simulink model "OMAP"  (R2018b)
settings: Solver=FixedStepDiscrete  StartTime=0.0  StopTime=10.0  FixedStep=0.01  RelTol=1e-3
values from neighbouring files (symbols this model uses):
  Clb_ICADirect_LaneDisp_StateFive = Simulink.Parameter    [omap_ver_442.m]
  Clb_ICADirect_LaneDisp_StateFour = Simulink.Parameter    [omap_ver_442.m]
  Clb_ICADirect_LaneDisp_StateOne = Simulink.Parameter    [omap_ver_442.m]
  Clb_ICADirect_LaneDisp_StateThree = Simulink.Parameter    [omap_ver_442.m]
  Clb_ICADirect_LaneDisp_StateTwo = Simulink.Parameter    [omap_ver_442.m]
  Clb_ICADirect_LaneDisp_StateZero = Simulink.Parameter    [omap_ver_442.m]
  Clb_ICADirect_LaneDispSW = Simulink.Parameter    [omap_ver_442.m]
  Clb_ICADirect_TrnLghtsCom_Switch = Simulink.Parameter    [omap_ver_442.m]
  Clb_ICADirect_TrnLghtsCom_Value = Simulink.Parameter    [omap_ver_442.m]
  Clb_ICADirect_TrnLghtsCrtl_Inhb = Simulink.Parameter    [omap_ver_442.m]
  OMAP_ACCAEB_EMSESC_Decel = Simulink.Parameter    [omap_ver_442.m]
  OMAP_ACCFCW_IC_Decel = Simulink.Parameter    [omap_ver_442.m]
  OMAP_clb_ACC_RVVReqType = Simulink.Parameter    [omap_ver_442.m]
  OMAP_clb_ACC_RVVReqType_Switch = Simulink.Parameter    [omap_ver_442.m]
  OMAP_clb_ACCHeadwayDisplay = Simulink.Parameter    [omap_ver_442.m]
  OMAP_clb_ACCHeadwayDisplay_Switch = Simulink.Parameter    [omap_ver_442.m]
  OMAP_clb_ACCHeadwayIcon = Simulink.Parameter    [omap_ver_442.m]
  OMAP_clb_ACCHeadwayIcon_Switch = Simulink.Parameter    [omap_ver_442.m]
  OMAP_clb_ACCMessagePrompt = Simulink.Parameter    [omap_ver_442.m]
  OMAP_clb_ACCMessagePrompt_Switch = Simulink.Parameter    [omap_ver_442.m]
  OMAP_clb_ACCRequestEPB = Simulink.Parameter    [omap_ver_442.m]
  OMAP_clb_ACCRequestEPB_Switch = Simulink.Parameter    [omap_ver_442.m]
  OMAP_clb_ACCSetSpeed = Simulink.Parameter    [omap_ver_442.m]
  OMAP_clb_ACCSetSpeed_Switch = Simulink.Parameter    [omap_ver_442.m]
  OMAP_clb_ACCSetSpeedDis = Simulink.Parameter    [omap_ver_442.m]
  OMAP_clb_ACCSetSpeedDis_Switch = Simulink.Parameter    [omap_ver_442.m]
  OMAP_clb_ACCState = Simulink.Parameter    [omap_ver_442.m]
  OMAP_clb_ACCState_Switch = Simulink.Parameter    [omap_ver_442.m]
  OMAP_clb_ACCStatusIconDis = Simulink.Parameter    [omap_ver_442.m]
  OMAP_clb_ACCStatusIconDis_Switch = Simulink.Parameter    [omap_ver_442.m]
  OMAP_clb_ACCTorqueReq = Simulink.Parameter    [omap_ver_442.m]
  OMAP_clb_ACCTorqueReq_Switch = Simulink.Parameter    [omap_ver_442.m]
  OMAP_clb_ADAS_State = Simulink.Parameter    [omap_ver_442.m]
  OMAP_clb_ADAS_State_Switch = Simulink.Parameter    [omap_ver_442.m]
  OMAP_clb_AEBAlertReq = Simulink.Parameter    [omap_ver_442.m]
  OMAP_clb_AEBAlertReq_Switch = Simulink.Parameter    [omap_ver_442.m]
  OMAP_clb_AEBBrakingProg = Simulink.Parameter    [omap_ver_442.m]
  OMAP_clb_AEBBrakingProg_Switch = Simulink.Parameter    [omap_ver_442.m]
  OMAP_clb_AEBFaultStatus = Simulink.Parameter    [omap_ver_442.m]
  OMAP_clb_AEBFaultStatus_Switch = Simulink.Parameter    [omap_ver_442.m]
  OMAP_clb_AEBMassageDisp = Simulink.Parameter    [omap_ver_442.m]
  OMAP_clb_AEBMassageDisp_Switch = Simulink.Parameter    [omap_ver_442.m]
  OMAP_clb_AEBState = Simulink.Parameter    [omap_ver_442.m]
  OMAP_clb_AEBState_Switch = Simulink.Parameter    [omap_ver_442.m]
  OMAP_clb_AEBSwitchStatus = Simulink.Parameter    [omap_ver_442.m]
  OMAP_clb_AEBSwitchStatus_Switch = Simulink.Parameter    [omap_ver_442.m]
  OMAP_clb_BrakeRequest = Simulink.Parameter    [omap_ver_442.m]
  OMAP_clb_BrakeRequest_Switch = Simulink.Parameter    [omap_ver_442.m]
  OMAP_clb_DecelerationSet = Simulink.Parameter    [omap_ver_442.m]
  OMAP_clb_DecelerationSet_Switch = Simulink.Parameter    [omap_ver_442.m]
  OMAP_clb_DecelerationType = Simulink.Parameter    [omap_ver_442.m]
  OMAP_clb_DecelerationType_Switch = Simulink.Parameter    [omap_ver_442.m]
  OMAP_clb_DeclControlReq = Simulink.Parameter    [omap_ver_442.m]
  OMAP_clb_DeclControlReq_Switch = Simulink.Parameter    [omap_ver_442.m]
  OMAP_clb_DownorUpGearMinTime = Simulink.Parameter    [omap_ver_442.m]
  OMAP_clb_DownorUpGearMinTime_Switch = Simulink.Parameter    [omap_ver_442.m]
  OMAP_clb_ELKPopupMessage = Simulink.Parameter    [omap_ver_442.m]
  OMAP_clb_ELKPopupMessage_Switch = Simulink.Parameter    [omap_ver_442.m]
  OMAP_clb_ELKSts = Simulink.Parameter    [omap_ver_442.m]
  OMAP_clb_ELKSts_Switch = Simulink.Parameter    [omap_ver_442.m]
  OMAP_clb_ESAFaultSt = Simulink.Parameter    [omap_ver_442.m]
  OMAP_clb_ESAFaultSt_Switch = Simulink.Parameter    [omap_ver_442.m]
  OMAP_clb_ESARequest = Simulink.Parameter    [omap_ver_442.m]
  OMAP_clb_ESARequest_Switch = Simulink.Parameter    [omap_ver_442.m]
  OMAP_clb_ESAState = Simulink.Parameter    [omap_ver_442.m]
  OMAP_clb_ESAState_Switch = Simulink.Parameter    [omap_ver_442.m]
  OMAP_clb_ESATorqueReq = Simulink.Parameter    [omap_ver_442.m]
  OMAP_clb_ESATorqueReq_Switch = Simulink.Parameter    [omap_ver_442.m]
  OMAP_clb_ESCDriveOff = Simulink.Parameter    [omap_ver_442.m]
  OMAP_clb_ESCDriveOff_Switch = Simulink.Parameter    [omap_ver_442.m]
  OMAP_clb_ESCHoldReq = Simulink.Parameter    [omap_ver_442.m]
  OMAP_clb_ESCHoldReq_Switch = Simulink.Parameter    [omap_ver_442.m]
  OMAP_clb_Handsoffwarning = Simulink.Parameter    [omap_ver_442.m]
  OMAP_clb_Handsoffwarning_Switch = Simulink.Parameter    [omap_ver_442.m]
  OMAP_clb_HapticAlarmReq = Simulink.Parameter    [omap_ver_442.m]
  OMAP_clb_HapticAlarmReq_Switch = Simulink.Parameter    [omap_ver_442.m]
  OMAP_clb_HMIPopupMassage = Simulink.Parameter    [omap_ver_442.m]
  OMAP_clb_HMIPopupMassage_Switch = Simulink.Parameter    [omap_ver_442.m]
  OMAP_clb_HWAActionSts = Simulink.Parameter    [omap_ver_442.m]
  OMAP_clb_HWAActionSts_Switch = Simulink.Parameter    [omap_ver_442.m]
  OMAP_clb_HWAMode = Simulink.Parameter    [omap_ver_442.m]
  OMAP_clb_HWAMode_Switch = Simulink.Parameter    [omap_ver_442.m]
  OMAP_clb_HWATurnOnIdctr = Simulink.Parameter    [omap_ver_442.m]
  OMAP_clb_HWATurnOnIdctr_Switch = Simulink.Parameter    [omap_ver_442.m]
  OMAP_clb_ICAMassageDisp = Simulink.Parameter    [omap_ver_442.m]
  OMAP_clb_ICAMassageDisp_Switch = Simulink.Parameter    [omap_ver_442.m]
  OMAP_clb_ICAStatusIcon = Simulink.Parameter    [omap_ver_442.m]
  OMAP_clb_ICAStatusIcon_Switch = Simulink.Parameter    [omap_ver_442.m]
  OMAP_clb_ISLCDriverRemind = Simulink.Parameter    [omap_ver_442.m]
  OMAP_clb_ISLCDriverRemind_Switch = Simulink.Parameter    [omap_ver_442.m]
  OMAP_clb_ISLCState = Simulink.Parameter    [omap_ver_442.m]
  OMAP_clb_ISLCState_Switch = Simulink.Parameter    [omap_ver_442.m]
  OMAP_clb_JAFaultSt = Simulink.Parameter    [omap_ver_442.m]
  OMAP_clb_JAFaultSt_Switch = Simulink.Parameter    [omap_ver_442.m]
  OMAP_clb_LCAPopupMessage = Simulink.Parameter    [omap_ver_442.m]
  OMAP_clb_LCAPopupMessage_Switch = Simulink.Parameter    [omap_ver_442.m]
  OMAP_clb_LCAStatusDisplay = Simulink.Parameter    [omap_ver_442.m]
  OMAP_clb_LCAStatusDisplay_Switch = Simulink.Parameter    [omap_ver_442.m]
  OMAP_clb_LDWStatusDisplay = Simulink.Parameter    [omap_ver_442.m]
  OMAP_clb_LDWStatusDisplay_Switch = Simulink.Parameter    [omap_ver_442.m]
  OMAP_clb_LDWWarningSt = Simulink.Parameter    [omap_ver_442.m]
  OMAP_clb_LDWWarningSt_Switch = Simulink.Parameter    [omap_ver_442.m]
  OMAP_clb_LightControlValid = Simulink.Parameter    [omap_ver_442.m]
  OMAP_clb_LightControlValid_Switch = Simulink.Parameter    [omap_ver_442.m]
  OMAP_clb_LKAActivation = Simulink.Parameter    [omap_ver_442.m]
  OMAP_clb_LKAActivation_Switch = Simulink.Parameter    [omap_ver_442.m]
  OMAP_clb_LKAAngleReq = Simulink.Parameter    [omap_ver_442.m]
  OMAP_clb_LKAAngleReq_Switch = Simulink.Parameter    [omap_ver_442.m]
  OMAP_clb_LKAMode = Simulink.Parameter    [omap_ver_442.m]
  OMAP_clb_LKAMode_Switch = Simulink.Parameter    [omap_ver_442.m]
  OMAP_clb_LKAorELK_CoolTime = Simulink.Parameter    [omap_ver_442.m]
  OMAP_clb_LKAState = Simulink.Parameter    [omap_ver_442.m]
  OMAP_clb_LKAState_Switch = Simulink.Parameter    [omap_ver_442.m]
  OMAP_clb_LKAStatusDisplay = Simulink.Parameter    [omap_ver_442.m]
  OMAP_clb_LKAStatusDisplay_Switch = Simulink.Parameter    [omap_ver_442.m]
  OMAP_clb_LKASwitchState = Simulink.Parameter    [omap_ver_442.m]
  OMAP_clb_LKASwitchState_Switch = Simulink.Parameter    [omap_ver_442.m]
  OMAP_clb_LKATorqFactReq = Simulink.Parameter    [omap_ver_442.m]
  OMAP_clb_LKATorqFactReq_Switch = Simulink.Parameter    [omap_ver_442.m]
  OMAP_clb_PrefillRequest = Simulink.Parameter    [omap_ver_442.m]
  ... (+36 more)
libraries: simulink x184, canmsglib x2
(part 12 of 14)

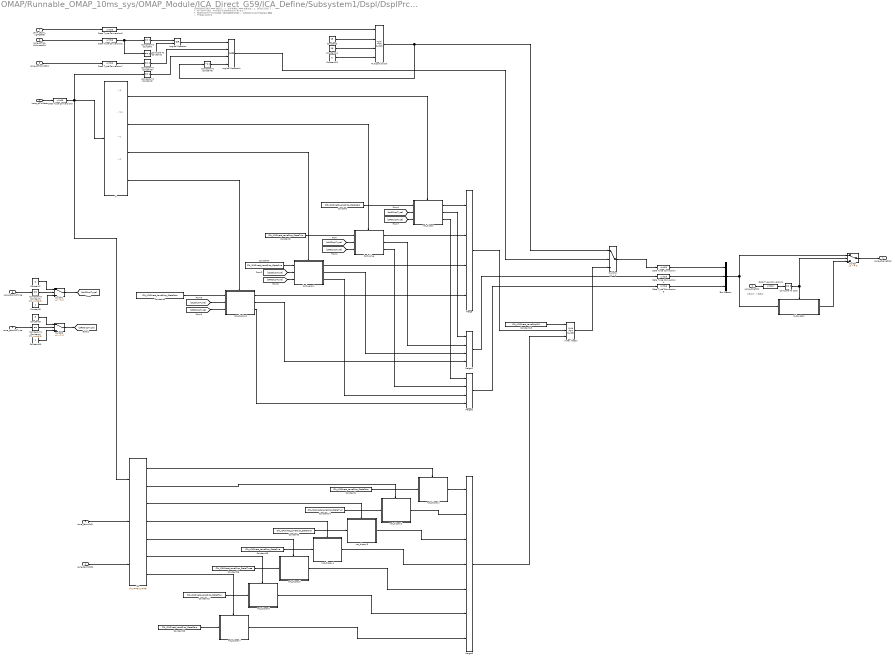
== system OMAP/Runnable_OMAP_10ms_sys/OMAP_Module/ICA_Direct_G59/ICA_Define/Subsystem1/Dspl/DsplPrcs/Lane ==
  note: 变道但条件不满足的车道线显示：
      | 1、多车道模式为TLC或者ALC；
      | 1、转向灯已经打了；
      | 2、由于条件不满足，THmode无法跳到状态4（=1或2）；
      | 3、驾驶员没有自己打方向变道（通过接管信号判断），此条其实可以由THState=3覆盖
      | 4、THState在状态3
  note: ->1
  note: ->14
  note: ->2
  note: ->0
  note: 0是运动，1是静止
  Lane_stTHState : Inport
  Lane_stVehSty : Inport  Port=2
  Lane_facmL0Ql : Inport  Port=3
  Lane_facmR0Ql : Inport  Port=4
  Lane_facmL0Type : Inport  Port=5
  Lane_facmR0Type : Inport  Port=6
  Lane_stturn_lightState : Inport  Port=7
  Lane_stTLC_ALCmodeSW : Inport  Port=8
  Lane_stTkOvStChk : Inport  Port=9
  Bus Creator : BusCreator  Inputs=3
  Compare To Constant : simulink/Logic and Bit Operations/Compare To Constant  relop===  const=2  OutDataTypeStr=boolean
  Compare To Constant1 : simulink/Logic and Bit Operations/Compare To Constant  relop===  const=3  OutDataTypeStr=boolean
  Compare To Constant2 : simulink/Logic and Bit Operations/Compare To Constant  relop===  const=3  OutDataTypeStr=boolean
  Compare To Constant3 : simulink/Logic and Bit Operations/Compare To Constant  relop===  const=uint16(3)  OutDataTypeStr=boolean
  Compare To Constant4 : simulink/Logic and Bit Operations/Compare To Constant  relop===  const=uint16(3)  OutDataTypeStr=boolean
  Compare To Constant5 : simulink/Logic and Bit Operations/Compare To Constant  relop===  const=0  OutDataTypeStr=boolean
  Compare To Constant6 : simulink/Logic and Bit Operations/Compare To Constant  relop=~=  const=0  OutDataTypeStr=boolean
  Compare To Zero : simulink/Logic and Bit Operations/Compare To Zero  relop===  OutDataTypeStr=boolean
  Constant{,1,5,13} (4 alike) : Constant  Value=Clb_ICADirect_LaneDisp_StateZero  OutDataTypeStr=uint16
  Constant10 : Constant  OutDataTypeStr=uint16
  Constant11 : Constant  Value=16  OutDataTypeStr=uint16
  Constant12 : Constant  Value=0  OutDataTypeStr=uint16
  Constant14 : Constant  Value=Clb_ICADirect_LaneDisp_StateTwo  OutDataTypeStr=uint16
  Constant15 : Constant  Value=Clb_ICADirect_LaneDisp_StateFive  OutDataTypeStr=uint16
  Constant16 : Constant  Value=Clb_ICADirect_LaneDisp_StateThree  OutDataTypeStr=uint16
  Constant17 : Constant  Value=Clb_ICADirect_LaneDisp_StateFour  OutDataTypeStr=uint16
  Constant18 : Constant  Value=Clb_ICADirect_LaneDispSW  OutDataTypeStr=boolean
  Constant2 : Constant  Value=Clb_ICADirect_LaneDisp_StateTwo  OutDataTypeStr=uint16
  Constant3 : Constant  Value=15  OutDataTypeStr=uint16
  Constant4 : Constant  Value=Clb_ICADirect_LaneDisp_StateOne  OutDataTypeStr=uint16
  Constant6 : Constant  Value=Clb_ICADirect_LaneDisp_StateOne  OutDataTypeStr=uint16
  Constant7 : Constant  Value=3  OutDataTypeStr=uint16
  Constant8 : Constant  OutDataTypeStr=uint16
  Constant9 : Constant  Value=3  OutDataTypeStr=uint16
  Data Type Conversion{,1..7} (8 alike) : DataTypeConversion  OutDataTypeStr=uint16
  If : If  IfExpression=u1==0|u1==5  ElseIfExpressions=u1==3,(u1==1|u1==2|u1==4|u1==6|u1==7|u1==8)
  If1 : If  NumInputs=3  IfExpression=u1==0|u1==5  ElseIfExpressions=u1==3,u1==1|u1==4|(u2<3&u3<3),u2==3&u3==3,u2==3&u3<3,u2<3&u3==3
  Index Vector : MultiPortSwitch  DataPortOrder=Zero-based contiguous  Inputs=2  zeroidx=on
  Logical Operator : Logic  Operator=OR  AllPortsSameDT=off  OutDataTypeStr=boolean
  Logical Operator1 : Logic  Inputs=4  AllPortsSameDT=off  OutDataTypeStr=boolean
  Merge : Merge  Inputs=4
  Merge1 : Merge  Inputs=4
  Merge2 : Merge  Inputs=4
  Merge3 : Merge  Inputs=7
  Multiport Switch : MultiPortSwitch  Inputs=2  DataPortIndices={1,2}  DataPortForDefault=Additional data port  DiagnosticForDefault=None
  Subsystem : Subsystem
  Switch : Switch  Criteria=u2 ~= 0
  Switch1 : Switch  Criteria=u2 ~= 0
  Switch2 : Switch  Criteria=u2 ~= 0
  Switch3 : Switch  Criteria=u2 > Threshold  OutDataTypeStr=uint16
  both_blue : Subsystem  TreatAsAtomicUnit=on
  both_gray1 : Subsystem  TreatAsAtomicUnit=on
  not_dispay : Subsystem  TreatAsAtomicUnit=on
  not_dispay1 : Subsystem  TreatAsAtomicUnit=on
  not_dispay2 : Subsystem  TreatAsAtomicUnit=on
  not_dispay3 : Subsystem  TreatAsAtomicUnit=on
  not_dispay4 : Subsystem  TreatAsAtomicUnit=on
  not_dispay5 : Subsystem  TreatAsAtomicUnit=on
  not_dispay6 : Subsystem  TreatAsAtomicUnit=on
  not_dispay7 : Subsystem  TreatAsAtomicUnit=on
  not_display2 : Subsystem  TreatAsAtomicUnit=on
  Lane_stLaneDspl : Outport
  wires:
  If/1 -> not_dispay/Action
  Lane_stVehSty/1 -> Data Type Conversion1/1
  both_gray1/1(Out1) -> Merge/3
  Lane_facmR0Type/1 -> Compare To Constant4/1
  Lane_facmR0Ql/1 -> If1/3
  Switch/1 -> Lane_stLaneDspl/1
  Compare To Zero/1 -> Switch/2, Subsystem/Enable
  Compare To Constant3/1 -> Switch1/2
  not_display2/1(Out1) -> Merge/4
  Lane_facmL0Type/1 -> Compare To Constant3/1
  Lane_facmL0Ql/1 -> If1/2
  Data Type Conversion5/1 -> Bus Creator/3  "stR0DispType"
  not_dispay/1(Out1) -> Merge/1
  [stL0DispType] -> both_blue/2(In2)
  Compare To Constant4/1 -> Switch2/2
  Constant2/1 -> both_blue/1(In1)
  both_blue/1(Out1) -> Merge/2
  Switch1/1 -> [stL0DispType]
  Subsystem/1(Out1) -> Switch/3
  [stR0DispType] -> both_blue/3(In3)
  Data Type Conversion4/1 -> Bus Creator/2  "stL0DispType"
  Constant8/1 -> Switch1/3
  Merge2/1 -> Data Type Conversion5/1
  Switch2/1 -> [stR0DispType]
  both_blue/3(Out3) -> Merge2/2
  Lane_stTHState/1 -> Data Type Conversion3/1
  Constant9/1 -> Switch2/1
  Merge1/1 -> Data Type Conversion4/1
  not_display2/3(Out3) -> Merge2/4
  Constant10/1 -> Switch2/3
  If/3 -> both_gray1/Action
  not_dispay/3(Out3) -> Merge2/1
  Constant7/1 -> Switch1/1
  If/2 -> both_blue/Action
  [stL0DispType] -> both_gray1/2(In2)
  If/4 -> not_display2/Action
  not_display2/2(Out2) -> Merge1/4
  Constant/1 -> not_dispay/1(In1)
  Bus Creator/1 -> Switch/1, Subsystem/1(In1)
  both_gray1/2(Out2) -> Merge1/3
  [stR0DispType] -> both_gray1/3(In3)
  Merge/1 -> Index Vector/2  "stLaneDspl"
  Data Type Conversion1/1 -> Compare To Zero/1
  [stR0DispType] -> not_dispay/3(In3)
  not_dispay/2(Out2) -> Merge1/1
  [stL0DispType] -> not_dispay/2(In2)
  [stL0DispType] -> not_display2/2(In2)
  Constant5/1 -> not_display2/1(In1)
  Constant4/1 -> both_gray1/1(In1)
  both_gray1/3(Out3) -> Merge2/3
  both_blue/2(Out2) -> Merge1/2
  [stR0DispType] -> not_display2/3(In3)
  Data Type Conversion/1 -> Bus Creator/1  "stLaneDspl"
  Switch3/1 -> Data Type Conversion/1
  Data Type Conversion2/1 -> Compare To Constant1/1, Compare To Constant/1
  Compare To Constant/1 -> Logical Operator/1
  Compare To Constant1/1 -> Logical Operator/2
  Lane_stTLC_ALCmodeSW/1 -> Data Type Conversion2/1
  Lane_stturn_lightState/1 -> Data Type Conversion6/1
  Lane_stTkOvStChk/1 -> Data Type Conversion7/1
  Data Type Conversion7/1 -> Compare To Constant5/1
  Constant3/1 -> Multiport Switch/2
  Constant11/1 -> Multiport Switch/3
  Constant12/1 -> Multiport Switch/4
  Data Type Conversion6/1 -> Multiport Switch/1
  Logical Operator/1 -> Logical Operator1/1
  Compare To Constant5/1 -> Logical Operator1/2
  Compare To Constant2/1 -> Logical Operator1/3
  Multiport Switch/1 -> Compare To Constant6/1, Switch3/1
  Compare To Constant6/1 -> Logical Operator1/4
  Logical Operator1/1 -> Switch3/2
  If1/1 -> not_dispay1/Action
  Constant1/1 -> not_dispay1/1(In1)
  Data Type Conversion3/1 -> If1/1, Compare To Constant2/1, If/1
  If1/2 -> not_dispay2/Action
  Constant14/1 -> not_dispay2/1(In1)
  If1/3 -> not_dispay3/Action
  Constant6/1 -> not_dispay3/1(In1)
  If1/4 -> not_dispay4/Action
  Constant15/1 -> not_dispay4/1(In1)
  If1/5 -> not_dispay5/Action
  Constant16/1 -> not_dispay5/1(In1)
  If1/6 -> not_dispay6/Action
  Constant17/1 -> not_dispay6/1(In1)
  If1/7 -> not_dispay7/Action
  Constant13/1 -> not_dispay7/1(In1)
  not_dispay1/1(Out1) -> Merge3/1
  not_dispay2/1(Out1) -> Merge3/2
  not_dispay3/1(Out1) -> Merge3/3
  not_dispay4/1(Out1) -> Merge3/4
  not_dispay5/1(Out1) -> Merge3/5
  not_dispay6/1(Out1) -> Merge3/6
  not_dispay7/1(Out1) -> Merge3/7
  Constant18/1 -> Index Vector/1
  Merge3/1 -> Index Vector/3  "stLaneDspl"
  Index Vector/1 -> Switch3/3

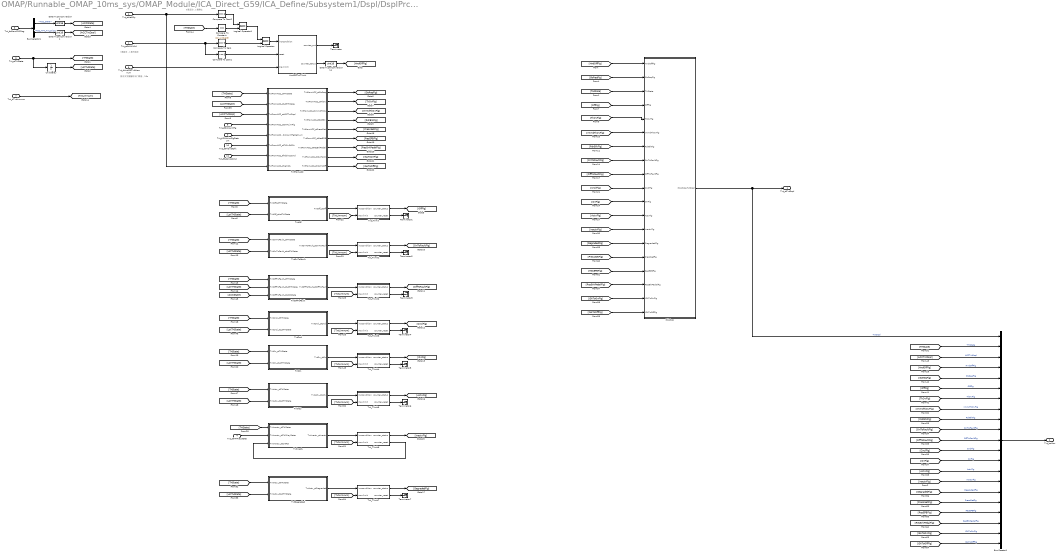
== system OMAP/Runnable_OMAP_10ms_sys/OMAP_Module/ICA_Direct_G59/ICA_Define/Subsystem1/Dspl/DsplPrcs/Txt ==
  note: 0是脱手，1是不脱手
  note: 脱手文字提醒时间门限值，15s
  note: 0是运动，1是静止
  Txt_stStWhlHld : Inport
  Txt_stVehSty : Inport  Port=2
  Txt_bsFromFMCMsg : Inport  Port=3
  Txt_stTHFKeyState : Inport  Port=4
  Txt_dHndOffTxtWarnnum : Inport  Port=5
  Txt_stTHState : Inport  Port=6
  Txt_dTxtLimnum : Inport  Port=7
  Txt_stSWALimFlg : Inport  Port=8
  Txt_tiSWALimFlgDetnum : Inport  Port=9
  Txt_stTkOvStChk : Inport  Port=10
  Txt_tfAddVocCmd : Inport  Port=11
  Bus Creator1 : BusCreator  Inputs=21
  Bus Selector1 : BusSelector  OutputSignals=ACC_State,ACC_HMI_Txt_Disp
  Compare To Constant : simulink/Logic and Bit Operations/Compare To Constant  relop===  const=uint16(3)  OutDataTypeStr=boolean
  Compare To Zero : simulink/Logic and Bit Operations/Compare To Zero  relop===  OutDataTypeStr=boolean
  Compare To Zero1 : simulink/Logic and Bit Operations/Compare To Zero  relop=~=  OutDataTypeStr=boolean
  Compare To Zero2 : simulink/Logic and Bit Operations/Compare To Zero  relop===  OutDataTypeStr=boolean
  Data Type Conversion1 : DataTypeConversion  OutDataTypeStr=uint16
  Data Type Conversion14 : DataTypeConversion  OutDataTypeStr=uint16
  Data Type Conversion2 : DataTypeConversion  OutDataTypeStr=uint16
  HndOffTxtTlimit : Subsystem
  Logical Operator : Logic  AllPortsSameDT=off  OutDataTypeStr=boolean
  Logical Operator1 : Logic  AllPortsSameDT=off  OutDataTypeStr=boolean
  PrioPrcs : MATLAB Function  TreatAsAtomicUnit=on
  Terminator{,1..7} (8 alike) : Terminator
  TxtActv : Subsystem
  TxtCncl : Subsystem
  TxtDegraded : Subsystem
  TxtFromACC : Subsystem
  TxtInactv : Subsystem
  TxtOff : Subsystem
  TxtOffToFault : Subsystem
  TxtOn : Subsystem
  TxtOnToFault : Subsystem
  Txt_Tlimit : Subsystem
  Txt_Tlimit1 : Subsystem
  Txt_Tlimit2 : Subsystem
  Txt_Tlimit3 : Subsystem
  Txt_Tlimit4 : Subsystem
  Txt_Tlimit5 : Subsystem
  Txt_Tlimit6 : Subsystem
  Txt_Tlimit7 : Subsystem
  Unit Delay : UnitDelay  SampleTime=-1
  Txt_stTxtDspl : Outport
  Txt_bsMon : Outport  Port=2
  wires:
  Compare To Zero/1 -> Logical Operator/2
  Txt_dHndOffTxtWarnnum/1 -> HndOffTxtTlimit/3(maxlimit)
  Compare To Zero1/1 -> HndOffTxtTlimit/2(reset)
  HndOffTxtTlimit/1(counter_out) -> Terminator/1
  Txt_stStWhlHld/1 -> Compare To Zero1/1, Compare To Zero/1
  HndOffTxtTlimit/2(counter_status) -> Data Type Conversion14/1
  [HndOffFlg] -> PrioPrcs/1(HndOffFlg)
  Txt_stTHState/1 -> Unit Delay/1, [THState]
  Unit Delay/1 -> [LstTHState]
  [THState] -> PrioPrcs/3(THState)
  [OffFlg] -> PrioPrcs/4(OffFlg)
  PrioPrcs/1(PrioPrcs_TxtDspl) -> Txt_stTxtDspl/1, Bus Creator1/1  "TxtDspl"
  [GoReqFlg] -> PrioPrcs/2(GoReqFlg)
  [TkOvFlg] -> PrioPrcs/5(TkOvFlg)
  [ImmdTkOvFlg] -> PrioPrcs/6(ImmdTkOvFlg)
  [RdrBlkFlg] -> PrioPrcs/7(RdrBlkFlg)
  [OnToFaultFlg] -> PrioPrcs/8(OnToFaultFlg)
  [OffToFaultFlg] -> PrioPrcs/9(OffToFaultFlg)
  [CnclFlg] -> PrioPrcs/10(CnclFlg)
  [OnFlg] -> PrioPrcs/11(OnFlg)
  [ActvFlg] -> PrioPrcs/12(ActvFlg)
  [InactvFlg] -> PrioPrcs/13(InactvFlg)
  [THState] -> Bus Creator1/2  "THState"
  [ACCTxtDspl] -> Bus Creator1/3  "ACCTxtDspl"
  [HndOffFlg] -> Bus Creator1/4  "HndOffFlg"
  [GoReqFlg] -> Bus Creator1/5  "GoReqFlg"
  [OffFlg] -> Bus Creator1/6  "OffFlg"
  [TkOvFlg] -> Bus Creator1/7  "TkOvFlg"
  [ImmdTkOvFlg] -> Bus Creator1/8  "ImmdTkOvFlg"
  [RdrBlkFlg] -> Bus Creator1/9  "RdrBlkFlg"
  [OnToFaultFlg] -> Bus Creator1/10  "OnToFaultFlg"
  [OffToFaultFlg] -> Bus Creator1/11  "OffToFaultFlg"
  [CnclFlg] -> Bus Creator1/12  "CnclFlg"
  [OnFlg] -> Bus Creator1/13  "OnFlg"
  [ActvFlg] -> Bus Creator1/14  "ActvFlg"
  [InactvFlg] -> Bus Creator1/15  "InactvFlg"
  Bus Creator1/1 -> Txt_bsMon/1
  Data Type Conversion14/1 -> [HndOffFlg]
  [THState] -> Compare To Constant/1
  Compare To Constant/1 -> Logical Operator1/2
  Logical Operator/1 -> HndOffTxtTlimit/1(incrcondition)
  Txt_bsFromFMCMsg/1 -> Bus Selector1/1
  Data Type Conversion1/1 -> [ACCTxtDspl]
  Bus Selector1/2 -> Data Type Conversion1/1  "<ACC_HMI_Txt_Disp>"
  Data Type Conversion2/1 -> [ACCState]
  Bus Selector1/1 -> Data Type Conversion2/1  "<ACC_State>"
  [THState] -> TxtOffToFault/1(TxtOffToFault_stTHState)
  [LstTHState] -> TxtOffToFault/2(TxtOffToFault_stLstTHState)
  [ACCState] -> TxtOffToFault/3(TxtOffToFault_stACCState)
  [LstTHState] -> TxtOnToFault/2(TxtOnToFault_stLstTHState)
  [THState] -> TxtOnToFault/1(TxtOnToFault_stTHState)
  [THState] -> TxtCncl/1(TxtCncl_stTHState)
  [LstTHState] -> TxtCncl/2(TxtCncl_stLstTHState)
  [LstTHState] -> TxtOn/2(TxtOn_stLstTHState)
  [THState] -> TxtOn/1(TxtOn_stTHState)
  [LstTHState] -> TxtActv/2(TxtActv_stLstTHState)
  [THState] -> TxtActv/1(TxtActv_stTHState)
  [THState] -> TxtInactv/1(TxtInactv_stTHState)
  Txt_stTHFKeyState/1 -> TxtInactv/2(TxtInactv_stTHFKeyState)
  [LstTHState] -> TxtOff/2(TxtOff_stLstTHState)
  [THState] -> TxtOff/1(TxtOff_stTHState)
  [THState] -> TxtFromACC/1(TxtFromACC_stTHState)
  [LstTHState] -> TxtFromACC/2(TxtFromACC_stLstTHState)
  [ACCTxtDspl] -> TxtFromACC/3(TxtFromACC_stACCTxtDspl)
  TxtFromACC/1(TxtFromACC_stGoReq) -> [GoReqFlg]
  TxtFromACC/2(TxtFromACC_stTkOv) -> [TkOvFlg]
  TxtFromACC/3(TxtFromACC_stImmdTkOv) -> [ImmdTkOvFlg]
  TxtFromACC/4(TxtFromACC_stRdrBlk) -> [RdrBlkFlg]
  Txt_dTxtLimnum/1 -> [TxtLimnum]
  [TxtLimnum] -> Txt_Tlimit/2(maxlimit)
  TxtOff/1(TxtOff_stOff) -> Txt_Tlimit/1(incrcondition)
  Txt_Tlimit/1(counter_status) -> [OffFlg]
  Txt_Tlimit1/1(counter_status) -> [OnToFaultFlg]
  TxtOnToFault/1(TxtOnToFault_stOnToFault) -> Txt_Tlimit1/1(incrcondition)
  [TxtLimnum] -> Txt_Tlimit1/2(maxlimit)
  [TxtLimnum] -> Txt_Tlimit2/2(maxlimit)
  TxtOffToFault/1(TxtOffToFault_stOffToFault) -> Txt_Tlimit2/1(incrcondition)
  Txt_Tlimit2/1(counter_status) -> [OffToFaultFlg]
  Txt_Tlimit3/1(counter_status) -> [CnclFlg]
  TxtCncl/1(TxtCncl_stCncl) -> Txt_Tlimit3/1(incrcondition)
  [TxtLimnum] -> Txt_Tlimit3/2(maxlimit)
  [TxtLimnum] -> Txt_Tlimit4/2(maxlimit)
  TxtOn/1(TxtOn_stOn) -> Txt_Tlimit4/1(incrcondition)
  Txt_Tlimit4/1(counter_status) -> [OnFlg]
  Txt_Tlimit5/1(counter_status) -> [ActvFlg]
  TxtActv/1(TxtActv_stActv) -> Txt_Tlimit5/1(incrcondition)
  [TxtLimnum] -> Txt_Tlimit5/2(maxlimit)
  [TxtLimnum] -> Txt_Tlimit6/2(maxlimit)
  TxtInactv/1(TxtInactv_stInactv) -> Txt_Tlimit6/1(incrcondition)
  Txt_Tlimit6/1(counter_status) -> [InactvFlg]
  Txt_Tlimit6/2(counter_reset) -> TxtInactv/3(TxtInactv_stCntRst)
  Txt_Tlimit/2(counter_reset) -> Terminator1/1
  Txt_Tlimit1/2(counter_reset) -> Terminator2/1
  Txt_Tlimit2/2(counter_reset) -> Terminator3/1
  Txt_Tlimit3/2(counter_reset) -> Terminator4/1
  Txt_Tlimit4/2(counter_reset) -> Terminator5/1
  Txt_Tlimit5/2(counter_reset) -> Terminator6/1
  Txt_stSWALimFlg/1 -> TxtFromACC/4(TxtFromACC_stSWALimFlg)
  Txt_tiSWALimFlgDetnum/1 -> TxtFromACC/5(TxtFromACC_tiSWALimFlgDetnum)
  Txt_stTkOvStChk/1 -> TxtFromACC/6(TxtFromACC_stTkOvStChk)
  Compare To Zero2/1 -> Logical Operator1/1
  Logical Operator1/1 -> Logical Operator/1
  [LstTHState] -> TxtDegraded/2(TxtActv_stLstTHState)
  [TxtLimnum] -> Txt_Tlimit7/2(maxlimit)
  Txt_Tlimit7/1(counter_status) -> [DegradedFlg]
  [THState] -> TxtDegraded/1(TxtActv_stTHState)
  TxtDegraded/1(TxtActv_stDegraded) -> Txt_Tlimit7/1(incrcondition)
  Txt_Tlimit7/2(counter_reset) -> Terminator7/1
  [DegradedFlg] -> Bus Creator1/16  "DegradedFlg"
  [DegradedFlg] -> PrioPrcs/14(DegradedFlg)
  TxtFromACC/5(TxtFromACC_stPressSet) -> [PressSetFlg]
  TxtFromACC/9(TxtFromACC_stISAToOff) -> [ISAToOffFlg]
  TxtFromACC/8(TxtFromACC_stISAToOn) -> [ISAToOnFlg]
  TxtFromACC/7(TxtFromACC_stResBrkPedal) -> [ResBrkPedalFlg]
  TxtFromACC/6(TxtFromACC_stResEPB) -> [ResEPBFlg]
  Txt_tfAddVocCmd/1 -> TxtFromACC/7(TxtFromACC_tfAddVocCmd)
  [ResBrkPedalFlg] -> PrioPrcs/17(ResBrkPedalFlg)
  [ISAToOnFlg] -> PrioPrcs/18(ISAToOnFlg)
  [ISAToOffFlg] -> PrioPrcs/19(ISAToOffFlg)
  [PressSetFlg] -> PrioPrcs/15(PressSetFlg)
  [ResEPBFlg] -> PrioPrcs/16(ResEPBFlg)
  [PressSetFlg] -> Bus Creator1/17  "PressSetFlg"
  [ResEPBFlg] -> Bus Creator1/18  "ResEPBFlg"
  [ResBrkPedalFlg] -> Bus Creator1/19  "ResBrkPedalFlg"
  [ISAToOnFlg] -> Bus Creator1/20  "ISAToOnFlg"
  [ISAToOffFlg] -> Bus Creator1/21  "ISAToOffFlg"
  Txt_stVehSty/1 -> TxtFromACC/8(TxtFromACC_stVehSty), Compare To Zero2/1

== system OMAP/Runnable_OMAP_10ms_sys/OMAP_Module/ICA_Direct_G59/ICA_Define/Subsystem1/Dspl/DsplPrcs/Voc ==
  note: 功能降级声音提示时长
  Voc_stStWhlHld : Inport
  Voc_stTHState : Inport  Port=2
  Voc_dDgrdVocWarnDurnum : Inport  Port=3
  Voc_dHndOffVocWarnnum : Inport  Port=4
  Voc_stVehSty : Inport  Port=5
  Compare To Constant : simulink/Logic and Bit Operations/Compare To Constant  relop===  const=uint16(3)  OutDataTypeStr=boolean
  Compare To Constant1 : simulink/Logic and Bit Operations/Compare To Constant  relop===  const=uint16(4)  OutDataTypeStr=boolean
  Compare To Constant2 : simulink/Logic and Bit Operations/Compare To Constant  relop===  const=uint16(3)  OutDataTypeStr=boolean
  Compare To Constant3 : simulink/Logic and Bit Operations/Compare To Constant  relop===  const=uint16(4)  OutDataTypeStr=boolean
  Compare To Zero1 : simulink/Logic and Bit Operations/Compare To Zero  relop===  OutDataTypeStr=boolean
  Compare To Zero2 : simulink/Logic and Bit Operations/Compare To Zero  relop===  OutDataTypeStr=boolean
  Data Type Conversion{,1..3} (4 alike) : DataTypeConversion  OutDataTypeStr=uint16
  Logical Operator : Logic  AllPortsSameDT=off  OutDataTypeStr=boolean
  Logical Operator1 : Logic  Inputs=3  AllPortsSameDT=off  OutDataTypeStr=boolean
  Logical Operator3 : Logic  Operator=OR  AllPortsSameDT=off  OutDataTypeStr=boolean
  MATLAB_Function : MATLAB Function  TreatAsAtomicUnit=on
  Sum_Condition : Subsystem  TreatAsAtomicUnit=on
  Switch : Switch  Criteria=u2 ~= 0
  Unit Delay : UnitDelay  SampleTime=-1
  Voc_stVocDspl : Outport
  wires:
  Voc_stTHState/1 -> Compare To Constant3/1, Compare To Constant2/1, Unit Delay/1, Compare To Constant1/1
  Unit Delay/1 -> Compare To Constant/1
  Compare To Constant1/1 -> Logical Operator/1
  Compare To Constant/1 -> Logical Operator/2
  Data Type Conversion/1 -> MATLAB_Function/1(Warning_duration)
  Data Type Conversion1/1 -> MATLAB_Function/2(Trigger)
  MATLAB_Function/1(Warning) -> Switch/2, Switch/1
  Voc_stStWhlHld/1 -> Compare To Zero1/1
  Sum_Condition/1(Out) -> Voc_stVocDspl/1
  Data Type Conversion3/1 -> Sum_Condition/Enable, Sum_Condition/1(In)
  Voc_dHndOffVocWarnnum/1 -> Data Type Conversion2/1
  Data Type Conversion2/1 -> Sum_Condition/2(Sum)
  Compare To Zero1/1 -> Logical Operator1/2
  Logical Operator1/1 -> Data Type Conversion3/1
  Voc_dDgrdVocWarnDurnum/1 -> Data Type Conversion/1
  Voc_stVehSty/1 -> Compare To Zero2/1
  Compare To Zero2/1 -> Logical Operator1/3
  Logical Operator/1 -> Data Type Conversion1/1
  Compare To Constant2/1 -> Logical Operator3/1
  Compare To Constant3/1 -> Logical Operator3/2
  Logical Operator3/1 -> Logical Operator1/1

== system OMAP/Runnable_OMAP_10ms_sys/OMAP_Module/Subsystem/EPS_Default_Arbitration/LKA_arb_ELK/Subsystem/Subsystem1/If Action Subsystem ==
  Action Port : ActionPort
  Constant : Constant  OutDataTypeStr=boolean
  Out1 : Outport
  wires:
  Constant/1 -> Out1/1

== system OMAP/Runnable_OMAP_10ms_sys/OMAP_Module/Subsystem/EPS_Default_Arbitration/LKA_arb_ELK/Subsystem/Subsystem1/If Action Subsystem1 ==
  In1 : Inport
  Action Port : ActionPort
  Out1 : Outport  OutDataTypeStr=boolean
  wires:
  In1/1 -> Out1/1

== system OMAP/Runnable_OMAP_10ms_sys/OMAP_Module/Subsystem/EPS_Default_Arbitration/LKA_arb_ELK/Subsystem/Subsystem1/If Action Subsystem2 ==
  Action Port : ActionPort
  Constant : Constant  Value=0  OutDataTypeStr=boolean
  Out1 : Outport
  wires:
  Constant/1 -> Out1/1

== system OMAP/Runnable_OMAP_10ms_sys/OMAP_Module/Subsystem/EPS_Default_Arbitration/LKA_arb_ELK/Subsystem/Subsystem1/Subsystem2 ==
  In1 : Inport
  Enable : EnablePort  StatesWhenEnabling=reset
  Add : Sum
  Constant : Constant  Value=0.01  OutDataTypeStr=single
  Memory : Memory  InheritSampleTime=on
  Relational Operator : RelationalOperator  Operator=<=  OutDataTypeStr=boolean  RndMeth=Simplest
  Saturation : Saturate  UpperLimit=5  LowerLimit=0
  Out1 : Outport
  wires:
  Memory/1 -> Add/2
  Saturation/1 -> Memory/1, Relational Operator/1
  Constant/1 -> Add/1
  Add/1 -> Saturation/1
  Relational Operator/1 -> Out1/1
  In1/1 -> Relational Operator/2

== system OMAP/Runnable_OMAP_10ms_sys/OMAP_Module/Subsystem/EPS_Default_Arbitration/LKA_arb_ELK/Subsystem/Subsystem2/If Action Subsystem ==
  Action Port : ActionPort
  Constant : Constant  OutDataTypeStr=boolean
  Out1 : Outport
  wires:
  Constant/1 -> Out1/1

== system OMAP/Runnable_OMAP_10ms_sys/OMAP_Module/Subsystem/EPS_Default_Arbitration/LKA_arb_ELK/Subsystem/Subsystem2/If Action Subsystem1 ==
  In1 : Inport
  Action Port : ActionPort
  Out1 : Outport  OutDataTypeStr=boolean
  wires:
  In1/1 -> Out1/1

== system OMAP/Runnable_OMAP_10ms_sys/OMAP_Module/Subsystem/EPS_Default_Arbitration/LKA_arb_ELK/Subsystem/Subsystem2/If Action Subsystem2 ==
  Action Port : ActionPort
  Constant : Constant  Value=0  OutDataTypeStr=boolean
  Out1 : Outport
  wires:
  Constant/1 -> Out1/1

== system OMAP/Runnable_OMAP_10ms_sys/OMAP_Module/Subsystem/EPS_Default_Arbitration/LKA_arb_ELK/Subsystem/Subsystem2/Subsystem2 ==
  In1 : Inport
  Enable : EnablePort  StatesWhenEnabling=reset
  Add : Sum
  Constant : Constant  Value=0.01  OutDataTypeStr=single
  Memory : Memory  InheritSampleTime=on
  Relational Operator : RelationalOperator  Operator=<=  OutDataTypeStr=boolean  RndMeth=Simplest
  Saturation : Saturate  UpperLimit=50  LowerLimit=0
  Out1 : Outport
  wires:
  In1/1 -> Relational Operator/2
  Relational Operator/1 -> Out1/1
  Add/1 -> Saturation/1
  Constant/1 -> Add/1
  Saturation/1 -> Relational Operator/1, Memory/1
  Memory/1 -> Add/2

== system OMAP/Runnable_OMAP_10ms_sys/OMAP_Module/Subsystem/ESC_Arbitration/ACC//ICA_arb_AEB//JA/AEB_arb_JA/AEB_arb_JA_STATUS/If Action Subsystem ==
  Action Port : ActionPort  ActionType=then
  Constant : Constant  Value=7  OutDataTypeStr=uint8
  Out1 : Outport
  wires:
  Constant/1 -> Out1/1

== system OMAP/Runnable_OMAP_10ms_sys/OMAP_Module/Subsystem/ESC_Arbitration/ACC//ICA_arb_AEB//JA/AEB_arb_JA/AEB_arb_JA_STATUS/If Action Subsystem1 ==
  Action Port : ActionPort  ActionType=elseif
  Constant : Constant  Value=3  OutDataTypeStr=uint8
  Out1 : Outport
  wires:
  Constant/1 -> Out1/1

== system OMAP/Runnable_OMAP_10ms_sys/OMAP_Module/Subsystem/ESC_Arbitration/ACC//ICA_arb_AEB//JA/AEB_arb_JA/AEB_arb_JA_STATUS/If Action Subsystem2 ==
  Action Port : ActionPort  ActionType=elseif
  Constant : Constant  Value=6  OutDataTypeStr=uint8
  Out1 : Outport
  wires:
  Constant/1 -> Out1/1

== system OMAP/Runnable_OMAP_10ms_sys/OMAP_Module/Subsystem/ESC_Arbitration/ACC//ICA_arb_AEB//JA/AEB_arb_JA/AEB_arb_JA_STATUS/If Action Subsystem3 ==
  Action Port : ActionPort  ActionType=elseif
  Constant : Constant  Value=5  OutDataTypeStr=uint8
  Out1 : Outport
  wires:
  Constant/1 -> Out1/1

== system OMAP/Runnable_OMAP_10ms_sys/OMAP_Module/Subsystem/ESC_Arbitration/ACC//ICA_arb_AEB//JA/AEB_arb_JA/AEB_arb_JA_STATUS/If Action Subsystem4 ==
  Action Port : ActionPort  ActionType=then
  Constant : Constant  Value=15  OutDataTypeStr=uint8
  Out1 : Outport
  wires:
  Constant/1 -> Out1/1

== system OMAP/Runnable_OMAP_10ms_sys/OMAP_Module/Subsystem/ESC_Arbitration/ACC//ICA_arb_AEB//JA/AEB_arb_JA/AEB_arb_JA_STATUS/If Action Subsystem5 ==
  Action Port : ActionPort  ActionType=elseif
  Constant : Constant  Value=6  OutDataTypeStr=uint8
  Out1 : Outport
  wires:
  Constant/1 -> Out1/1

== system OMAP/Runnable_OMAP_10ms_sys/OMAP_Module/Subsystem/ESC_Arbitration/ACC//ICA_arb_AEB//JA/AEB_arb_JA/AEB_arb_JA_STATUS/If Action Subsystem6 ==
  In1 : Inport
  Action Port : ActionPort  ActionType=else
  Data Type Conversion : DataTypeConversion  OutDataTypeStr=uint8
  Out1 : Outport  OutDataTypeStr=uint8
  wires:
  In1/1 -> Data Type Conversion/1
  Data Type Conversion/1 -> Out1/1

== system OMAP/Runnable_OMAP_10ms_sys/OMAP_Module/Subsystem/ESC_Arbitration/ACC//ICA_arb_AEB//JA/AEB_arb_JA/AEB_arb_JA_STATUS/If Action Subsystem7 ==
  Action Port : ActionPort  ActionType=elseif
  Constant : Constant  Value=12  OutDataTypeStr=uint8
  Out1 : Outport
  wires:
  Constant/1 -> Out1/1

== system OMAP/Runnable_OMAP_10ms_sys/OMAP_Module/Subsystem/ESC_Arbitration/ACC//ICA_arb_AEB//JA/AEB_arb_JA/AEB_arb_JA_STATUS/If Action Subsystem8 ==
  Action Port : ActionPort  ActionType=elseif
  Constant : Constant  Value=10  OutDataTypeStr=uint8
  Out1 : Outport
  wires:
  Constant/1 -> Out1/1

== system OMAP/Runnable_OMAP_10ms_sys/OMAP_Module/Subsystem/ESC_Arbitration/ACC//ICA_arb_AEB//JA/AEB_arb_JA/AEB_arb_JA_STATUS/If Action Subsystem9 ==
  In1 : Inport
  Action Port : ActionPort  ActionType=else
  Data Type Conversion : DataTypeConversion  OutDataTypeStr=uint8
  Out1 : Outport  OutDataTypeStr=uint8
  wires:
  In1/1 -> Data Type Conversion/1
  Data Type Conversion/1 -> Out1/1

== system OMAP/Runnable_OMAP_10ms_sys/OMAP_Module/ICA_Direct_G59/ICA_Define/Subsystem1/Dspl/DsplPrcs/Icon/If Action Subsystem ==
  In1 : Inport
  Action Port : ActionPort  ActionType=then
  Out1 : Outport
  wires:
  In1/1 -> Out1/1

== system OMAP/Runnable_OMAP_10ms_sys/OMAP_Module/ICA_Direct_G59/ICA_Define/Subsystem1/Dspl/DsplPrcs/Icon/If Action Subsystem1 ==
  In1 : Inport
  Action Port : ActionPort  ActionType=elseif
  Out1 : Outport
  wires:
  In1/1 -> Out1/1

== system OMAP/Runnable_OMAP_10ms_sys/OMAP_Module/ICA_Direct_G59/ICA_Define/Subsystem1/Dspl/DsplPrcs/Icon/If Action Subsystem10 ==
  In1 : Inport
  Action Port : ActionPort  ActionType=elseif
  Out1 : Outport
  wires:
  In1/1 -> Out1/1

== system OMAP/Runnable_OMAP_10ms_sys/OMAP_Module/ICA_Direct_G59/ICA_Define/Subsystem1/Dspl/DsplPrcs/Icon/If Action Subsystem11 ==
  In1 : Inport
  Action Port : ActionPort  ActionType=elseif
  Out1 : Outport
  wires:
  In1/1 -> Out1/1

== system OMAP/Runnable_OMAP_10ms_sys/OMAP_Module/ICA_Direct_G59/ICA_Define/Subsystem1/Dspl/DsplPrcs/Icon/If Action Subsystem12 ==
  In1 : Inport
  Action Port : ActionPort  ActionType=elseif
  Out1 : Outport
  wires:
  In1/1 -> Out1/1

== system OMAP/Runnable_OMAP_10ms_sys/OMAP_Module/ICA_Direct_G59/ICA_Define/Subsystem1/Dspl/DsplPrcs/Icon/If Action Subsystem13 ==
  In1 : Inport
  Action Port : ActionPort  ActionType=elseif
  Out1 : Outport
  wires:
  In1/1 -> Out1/1

== system OMAP/Runnable_OMAP_10ms_sys/OMAP_Module/ICA_Direct_G59/ICA_Define/Subsystem1/Dspl/DsplPrcs/Icon/If Action Subsystem14 ==
  In1 : Inport
  Action Port : ActionPort  ActionType=elseif
  Out1 : Outport
  wires:
  In1/1 -> Out1/1

== system OMAP/Runnable_OMAP_10ms_sys/OMAP_Module/ICA_Direct_G59/ICA_Define/Subsystem1/Dspl/DsplPrcs/Icon/If Action Subsystem15 ==
  In1 : Inport
  Action Port : ActionPort  ActionType=else
  Out1 : Outport
  wires:
  In1/1 -> Out1/1

== system OMAP/Runnable_OMAP_10ms_sys/OMAP_Module/ICA_Direct_G59/ICA_Define/Subsystem1/Dspl/DsplPrcs/Icon/If Action Subsystem16 ==
  In1 : Inport
  Action Port : ActionPort  ActionType=elseif
  Out1 : Outport
  wires:
  In1/1 -> Out1/1

== system OMAP/Runnable_OMAP_10ms_sys/OMAP_Module/ICA_Direct_G59/ICA_Define/Subsystem1/Dspl/DsplPrcs/Icon/If Action Subsystem2 ==
  In1 : Inport
  Action Port : ActionPort  ActionType=elseif
  Out1 : Outport
  wires:
  In1/1 -> Out1/1

== system OMAP/Runnable_OMAP_10ms_sys/OMAP_Module/ICA_Direct_G59/ICA_Define/Subsystem1/Dspl/DsplPrcs/Icon/If Action Subsystem3 ==
  In1 : Inport
  Action Port : ActionPort  ActionType=elseif
  Out1 : Outport
  wires:
  In1/1 -> Out1/1

== system OMAP/Runnable_OMAP_10ms_sys/OMAP_Module/ICA_Direct_G59/ICA_Define/Subsystem1/Dspl/DsplPrcs/Icon/If Action Subsystem4 ==
  In1 : Inport
  Action Port : ActionPort  ActionType=elseif
  Out1 : Outport
  wires:
  In1/1 -> Out1/1

== system OMAP/Runnable_OMAP_10ms_sys/OMAP_Module/ICA_Direct_G59/ICA_Define/Subsystem1/Dspl/DsplPrcs/Icon/If Action Subsystem5 ==
  In1 : Inport
  Action Port : ActionPort  ActionType=else
  Out1 : Outport
  wires:
  In1/1 -> Out1/1

== system OMAP/Runnable_OMAP_10ms_sys/OMAP_Module/ICA_Direct_G59/ICA_Define/Subsystem1/Dspl/DsplPrcs/Icon/If Action Subsystem6 ==
  In1 : Inport
  Action Port : ActionPort  ActionType=then
  Out1 : Outport
  wires:
  In1/1 -> Out1/1

== system OMAP/Runnable_OMAP_10ms_sys/OMAP_Module/ICA_Direct_G59/ICA_Define/Subsystem1/Dspl/DsplPrcs/Icon/If Action Subsystem7 ==
  In1 : Inport
  Action Port : ActionPort  ActionType=elseif
  Out1 : Outport
  wires:
  In1/1 -> Out1/1

== system OMAP/Runnable_OMAP_10ms_sys/OMAP_Module/ICA_Direct_G59/ICA_Define/Subsystem1/Dspl/DsplPrcs/Icon/If Action Subsystem8 ==
  In1 : Inport
  Action Port : ActionPort  ActionType=elseif
  Out1 : Outport
  wires:
  In1/1 -> Out1/1

== system OMAP/Runnable_OMAP_10ms_sys/OMAP_Module/ICA_Direct_G59/ICA_Define/Subsystem1/Dspl/DsplPrcs/Icon/If Action Subsystem9 ==
  In1 : Inport
  Action Port : ActionPort  ActionType=elseif
  Out1 : Outport
  wires:
  In1/1 -> Out1/1

== system OMAP/Runnable_OMAP_10ms_sys/OMAP_Module/ICA_Direct_G59/ICA_Define/Subsystem1/Dspl/DsplPrcs/Icon/else ==
  HiDurnum : Inport
  LoDurnum : Inport  Port=2
  Action Port : ActionPort  InitializeStates=reset  ActionType=else
  Add : Sum
  Constant1 : Constant  Value=0  OutDataTypeStr=uint16
  Constant8 : Constant  OutDataTypeStr=uint16
  Relational Operator1 : RelationalOperator  Operator=<=  OutDataTypeStr=boolean  RndMeth=Nearest
  Relational Operator2 : RelationalOperator  Operator=<=  OutDataTypeStr=boolean  RndMeth=Nearest
  Sum : Sum  OutDataTypeStr=Inherit: Inherit via back propagation  InputSameDT=on
  Unit Delay1 : UnitDelay  SampleTime=-1
  Unit Delay2 : UnitDelay  SampleTime=-1
  reset switch1 : Switch  Criteria=u2 ~= 0  Threshold=1  OutDataTypeStr=Inherit: Inherit via back propagation  InputSameDT=on
  count : Outport
  counter_status : Outport  Port=2
  wires:
  Unit Delay2/1 -> Sum/2
  Constant8/1 -> Sum/1
  Sum/1 -> reset switch1/3
  [reset] -> reset switch1/2
  Constant1/1 -> reset switch1/1
  Relational Operator1/1 -> Unit Delay1/1
  Unit Delay1/1 -> [reset]
  reset switch1/1 -> Unit Delay2/1, Relational Operator1/2, Relational Operator2/1, count/1
  Relational Operator2/1 -> counter_status/1
  Add/1 -> Relational Operator1/1
  LoDurnum/1 -> Add/2
  HiDurnum/1 -> Add/1, Relational Operator2/2

== system OMAP/Runnable_OMAP_10ms_sys/OMAP_Module/ICA_Direct_G59/ICA_Define/Subsystem1/Dspl/DsplPrcs/Icon/if ==
  In1 : Inport
  Action Port : ActionPort  ActionType=then
  Out1 : Outport
  wires:
  In1/1 -> Out1/1

== system OMAP/Runnable_OMAP_10ms_sys/OMAP_Module/ICA_Direct_G59/ICA_Define/Subsystem1/Dspl/DsplPrcs/Lane/Subsystem ==
  In1 : Inport
  Enable : EnablePort
  Out1 : Outport
  wires:
  In1/1 -> Out1/1

== system OMAP/Runnable_OMAP_10ms_sys/OMAP_Module/ICA_Direct_G59/ICA_Define/Subsystem1/Dspl/DsplPrcs/Lane/both_blue ==
  In1 : Inport
  In2 : Inport  Port=2
  In3 : Inport  Port=3
  Action Port : ActionPort  ActionType=elseif
  Out1 : Outport
  Out2 : Outport  Port=2
  Out3 : Outport  Port=3
  wires:
  In1/1 -> Out1/1
  In2/1 -> Out2/1
  In3/1 -> Out3/1

== system OMAP/Runnable_OMAP_10ms_sys/OMAP_Module/ICA_Direct_G59/ICA_Define/Subsystem1/Dspl/DsplPrcs/Lane/both_gray1 ==
  In1 : Inport
  In2 : Inport  Port=2
  In3 : Inport  Port=3
  Action Port : ActionPort  ActionType=elseif
  Out1 : Outport
  Out2 : Outport  Port=2
  Out3 : Outport  Port=3
  wires:
  In3/1 -> Out3/1
  In2/1 -> Out2/1
  In1/1 -> Out1/1

== system OMAP/Runnable_OMAP_10ms_sys/OMAP_Module/ICA_Direct_G59/ICA_Define/Subsystem1/Dspl/DsplPrcs/Lane/not_dispay ==
  In1 : Inport
  In2 : Inport  Port=2
  In3 : Inport  Port=3
  Action Port : ActionPort  ActionType=then
  Out1 : Outport
  Out2 : Outport  Port=2
  Out3 : Outport  Port=3
  wires:
  In3/1 -> Out3/1
  In2/1 -> Out2/1
  In1/1 -> Out1/1

== system OMAP/Runnable_OMAP_10ms_sys/OMAP_Module/ICA_Direct_G59/ICA_Define/Subsystem1/Dspl/DsplPrcs/Lane/not_dispay1 ==
  In1 : Inport
  Action Port : ActionPort  ActionType=then
  Out1 : Outport
  wires:
  In1/1 -> Out1/1

== system OMAP/Runnable_OMAP_10ms_sys/OMAP_Module/ICA_Direct_G59/ICA_Define/Subsystem1/Dspl/DsplPrcs/Lane/not_dispay2 ==
  In1 : Inport
  Action Port : ActionPort  ActionType=elseif
  Out1 : Outport
  wires:
  In1/1 -> Out1/1

== system OMAP/Runnable_OMAP_10ms_sys/OMAP_Module/ICA_Direct_G59/ICA_Define/Subsystem1/Dspl/DsplPrcs/Lane/not_dispay3 ==
  In1 : Inport
  Action Port : ActionPort  ActionType=elseif
  Out1 : Outport
  wires:
  In1/1 -> Out1/1

== system OMAP/Runnable_OMAP_10ms_sys/OMAP_Module/ICA_Direct_G59/ICA_Define/Subsystem1/Dspl/DsplPrcs/Lane/not_dispay4 ==
  In1 : Inport
  Action Port : ActionPort  ActionType=elseif
  Out1 : Outport
  wires:
  In1/1 -> Out1/1

== system OMAP/Runnable_OMAP_10ms_sys/OMAP_Module/ICA_Direct_G59/ICA_Define/Subsystem1/Dspl/DsplPrcs/Lane/not_dispay5 ==
  In1 : Inport
  Action Port : ActionPort  ActionType=elseif
  Out1 : Outport
  wires:
  In1/1 -> Out1/1

== system OMAP/Runnable_OMAP_10ms_sys/OMAP_Module/ICA_Direct_G59/ICA_Define/Subsystem1/Dspl/DsplPrcs/Lane/not_dispay6 ==
  In1 : Inport
  Action Port : ActionPort  ActionType=elseif
  Out1 : Outport
  wires:
  In1/1 -> Out1/1

== system OMAP/Runnable_OMAP_10ms_sys/OMAP_Module/ICA_Direct_G59/ICA_Define/Subsystem1/Dspl/DsplPrcs/Lane/not_dispay7 ==
  In1 : Inport
  Action Port : ActionPort  ActionType=else
  Out1 : Outport
  wires:
  In1/1 -> Out1/1

== system OMAP/Runnable_OMAP_10ms_sys/OMAP_Module/ICA_Direct_G59/ICA_Define/Subsystem1/Dspl/DsplPrcs/Lane/not_display2 ==
  In1 : Inport
  In2 : Inport  Port=2
  In3 : Inport  Port=3
  Action Port : ActionPort  ActionType=else
  Out1 : Outport
  Out2 : Outport  Port=2
  Out3 : Outport  Port=3
  wires:
  In1/1 -> Out1/1
  In2/1 -> Out2/1
  In3/1 -> Out3/1

== system OMAP/Runnable_OMAP_10ms_sys/OMAP_Module/ICA_Direct_G59/ICA_Define/Subsystem1/Dspl/DsplPrcs/Txt/HndOffTxtTlimit ==
  incrcondition : Inport
  reset : Inport  Port=2
  maxlimit : Inport  Port=3
  Constant : Constant  Value=0  OutDataTypeStr=uint16
  Constant1 : Constant  OutDataTypeStr=uint16
  Constant2 : Constant  Value=0  OutDataTypeStr=uint16
  Constant3 : Constant  Value=0  OutDataTypeStr=uint16
  MinMax1 : MinMax  Inputs=2  OutDataTypeStr=Inherit: Inherit via back propagation  InputSameDT=on
  MinMax2 : MinMax  Function=max  Inputs=2  OutDataTypeStr=Inherit: Inherit via back propagation  InputSameDT=on
  Relational Operator : RelationalOperator  OutDataTypeStr=boolean  RndMeth=Nearest
  Sum : Sum  OutDataTypeStr=Inherit: Inherit via back propagation  InputSameDT=on
  Unit Delay : UnitDelay  SampleTime=-1
  inc switch : Switch  Criteria=u2 ~= 0  Threshold=1  OutDataTypeStr=Inherit: Inherit via back propagation  InputSameDT=on
  reset switch : Switch  Criteria=u2 ~= 0  Threshold=1  OutDataTypeStr=Inherit: Inherit via back propagation  InputSameDT=on
  counter_out : Outport
  counter_status : Outport  Port=2
  wires:
  Relational Operator/1 -> counter_status/1
  reset switch/1 -> counter_out/1, Unit Delay/1, Relational Operator/1
  Constant2/1 -> MinMax2/1
  incrcondition/1 -> inc switch/2
  maxlimit/1 -> Relational Operator/2, MinMax1/2
  MinMax2/1 -> MinMax1/1
  Constant/1 -> inc switch/3
  Constant1/1 -> inc switch/1
  MinMax1/1 -> reset switch/3
  reset/1 -> reset switch/2
  Sum/1 -> MinMax2/2
  inc switch/1 -> Sum/2
  Constant3/1 -> reset switch/1
  Unit Delay/1 -> Sum/1

== system OMAP/Runnable_OMAP_10ms_sys/OMAP_Module/ICA_Direct_G59/ICA_Define/Subsystem1/Dspl/DsplPrcs/Txt/TxtActv ==
  TxtActv_stTHState : Inport
  TxtActv_stLstTHState : Inport  Port=2
  Constant1 : Constant  OutDataTypeStr=uint16
  Constant2 : Constant  Value=0  OutDataTypeStr=uint16
  Hold : Subsystem  TreatAsAtomicUnit=on
  If : If  NumInputs=2  IfExpression=(u1 == 3 |u1 == 4 |u1 == 6) & u2 == 2  ElseIfExpressions=u1 ~= 3 & u1 ~= 4 & u1 ~= 6
  Merge : Merge  Inputs=3
  Start : Subsystem  TreatAsAtomicUnit=on
  Stop : Subsystem  TreatAsAtomicUnit=on
  Unit Delay1 : UnitDelay  SampleTime=-1
  TxtActv_stActv : Outport
  wires:
  TxtActv_stTHState/1 -> If/1
  Merge/1 -> Unit Delay1/1, TxtActv_stActv/1
  Start/1(Out1) -> Merge/1
  TxtActv_stLstTHState/1 -> If/2
  Constant1/1 -> Start/1(In1)
  If/1 -> Start/Action
  Constant2/1 -> Stop/1(In1)
  If/2 -> Stop/Action
  Unit Delay1/1 -> Hold/1(In1)
  If/3 -> Hold/Action
  Stop/1(Out1) -> Merge/2
  Hold/1(Out1) -> Merge/3

== system OMAP/Runnable_OMAP_10ms_sys/OMAP_Module/ICA_Direct_G59/ICA_Define/Subsystem1/Dspl/DsplPrcs/Txt/TxtCncl ==
  TxtCncl_stTHState : Inport
  TxtCncl_stLstTHState : Inport  Port=2
  Constant1 : Constant  OutDataTypeStr=uint16
  Constant2 : Constant  Value=0  OutDataTypeStr=uint16
  Hold : Subsystem  TreatAsAtomicUnit=on
  If : If  NumInputs=2  IfExpression=u1 == 1 & (u2 == 3 | u2 == 4 | u2 == 6)  ElseIfExpressions=u1 ~= 1 & u1 ~= 2
  Merge : Merge  Inputs=3
  Start : Subsystem  TreatAsAtomicUnit=on
  Stop : Subsystem  TreatAsAtomicUnit=on
  Unit Delay1 : UnitDelay  SampleTime=-1
  TxtCncl_stCncl : Outport
  wires:
  Hold/1(Out1) -> Merge/3
  Stop/1(Out1) -> Merge/2
  If/3 -> Hold/Action
  Unit Delay1/1 -> Hold/1(In1)
  If/2 -> Stop/Action
  Constant2/1 -> Stop/1(In1)
  If/1 -> Start/Action
  Constant1/1 -> Start/1(In1)
  TxtCncl_stLstTHState/1 -> If/2
  Start/1(Out1) -> Merge/1
  Merge/1 -> TxtCncl_stCncl/1, Unit Delay1/1
  TxtCncl_stTHState/1 -> If/1

== system OMAP/Runnable_OMAP_10ms_sys/OMAP_Module/ICA_Direct_G59/ICA_Define/Subsystem1/Dspl/DsplPrcs/Txt/TxtDegraded ==
  TxtActv_stTHState : Inport
  TxtActv_stLstTHState : Inport  Port=2
  Constant1 : Constant  OutDataTypeStr=uint16
  Constant2 : Constant  Value=0  OutDataTypeStr=uint16
  Hold : Subsystem  TreatAsAtomicUnit=on
  If : If  NumInputs=2  IfExpression=u1 == 4 & u2 == 4  ElseIfExpressions=u1 ~= 4 & u2 == 4
  Merge : Merge  Inputs=3
  Start : Subsystem  TreatAsAtomicUnit=on
  Stop : Subsystem  TreatAsAtomicUnit=on
  Unit Delay1 : UnitDelay  SampleTime=-1
  TxtActv_stDegraded : Outport
  wires:
  TxtActv_stTHState/1 -> If/1
  Merge/1 -> Unit Delay1/1, TxtActv_stDegraded/1
  Start/1(Out1) -> Merge/1
  TxtActv_stLstTHState/1 -> If/2
  Constant1/1 -> Start/1(In1)
  If/1 -> Start/Action
  Constant2/1 -> Stop/1(In1)
  If/2 -> Stop/Action
  Unit Delay1/1 -> Hold/1(In1)
  If/3 -> Hold/Action
  Stop/1(Out1) -> Merge/2
  Hold/1(Out1) -> Merge/3
